simulink model "p4_v4"  (R2023b)
settings: Solver=VariableStepAuto  StartTime=0.0  StopTime=3600  RelTol=1e-3
values from neighbouring files (symbols this model uses):
  rps2rpm = 60/(2*pi())    [P4init.m]
undefined symbols (not defined in the file or in its folder): batData, carData, motorData
libraries: slpidlib x1
settings Model: Creator=lpoir  LastModifiedBy=lpoir

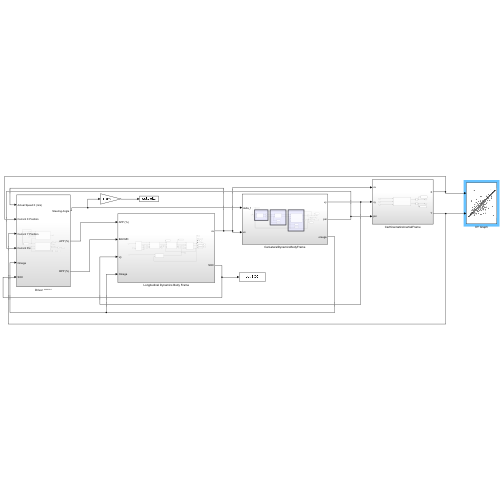
[thumbnail: Simulink's stored preview of the top-level diagram]
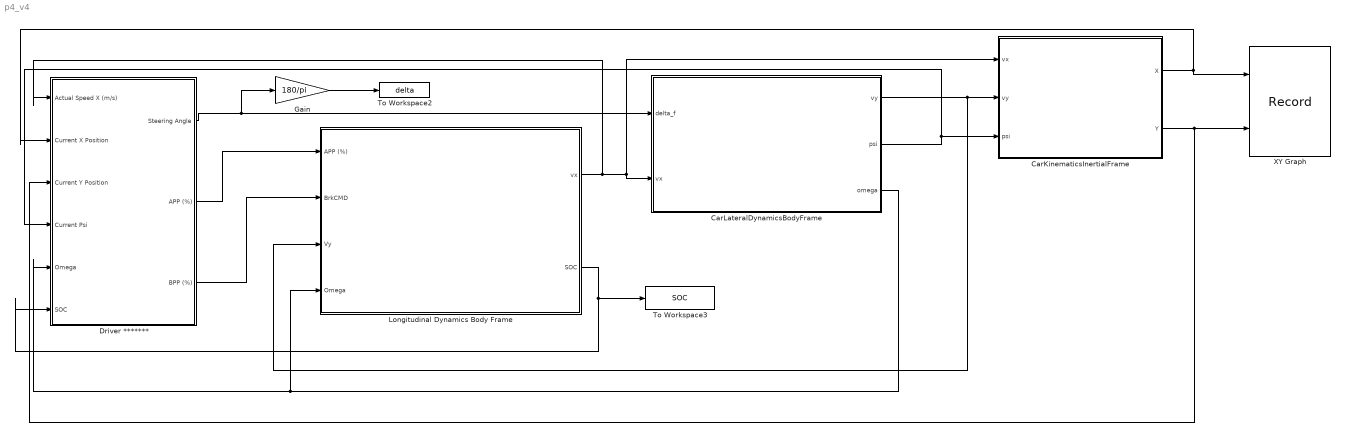
== system p4_v4 ==
  CarKinematicsInertialFrame : Subsystem
  CarLateralDynamicsBodyFrame : Subsystem
  Driver ******* : Subsystem
  Gain : Gain  Gain=180/pi
  Longitudinal Dynamics Body Frame : Subsystem
  To Workspace2 : ToWorkspace  VariableName=delta  SaveFormat=Timeseries  SampleTime=-1
  To Workspace3 : ToWorkspace  VariableName=SOC  SaveFormat=Timeseries  SampleTime=-1
  XY Graph : Record  FileSettingsInternal="{\"entries\":[{\"content\":{\"excelSettings\":{\"content\":{},\"type\":\"Streamout.ExcelSettings\"}},\"type\":\"Streamout.FileSettingStorage\",\"uuid\":\"\"}],\"packageUris\":[\"http:\\/\\/schema.mathworks.com\\/mf0\\/streamout_blocks\\/R2020a\"],\"version\":\"1.0\"}"  Layout=[1 1]  SignalsInternal="{\"entries\":[{\"content\":{\"signals\":[{\"content\":{\"blockPath\":[],\"dimensions\":[1],\"domain\":\"\",\"lineColor\":\"#a2142f\",\"plots\":[1],\"port\":1,\"sid\":[\"\"],\"signalID\":167009,\"signalName\":\"CarKinematicsInertialFrame:1\"},\"type\":\"RecordBlkView.Signal\",\"uuid\":\"\"},{\"content\":{\"blockPath\":[],\"dimensions\":[1],\"domain\":\"\",\"lineColor\":\"#139fff\",\"plots\":[1],\"port\":2,\"sid\":[\"\"],\"signalID\":167013,\"signalName\":\"CarKinematicsInertialFrame:2\"},\"type\":\"RecordBlkView.Signal\",\"uuid\":\"\"}]},\"type\":\"RecordBlkView.InputSignals\",\"uuid\":\"\"}],\"packageUris\":[\"http:\\/\\/schema.mathworks.com\\/mf0\\/streamout_blocks\\/R2020a\"],\"version\":\"1.0\"}"  VisualizationBindings="{\"xyplotplugin\":{\"info\":[{\"series\":[{\"bindingParametersList\":[{\"parameter\":\"X-Axis\",\"signalID\":167009,\"signalName\":\"CarKinematicsInertialFrame:1\"},{\"parameter\":\"Y-Axis\",\"signalID\":167013,\"signalName\":\"CarKinematicsInertialFrame:2\"}],\"seriesID\":48033}],\"subplotID\":1}]}}"  CompatibilityTag=XY
  wires:
  CarKinematicsInertialFrame/1(X) -> XY Graph/1, Driver *******/2(Current X Position)
  CarKinematicsInertialFrame/2(Y) -> XY Graph/2, Driver *******/3(Current Y Position)
  CarLateralDynamicsBodyFrame/2(psi) -> Driver *******/4("Current Psi "), CarKinematicsInertialFrame/3(psi)
  Longitudinal Dynamics Body Frame/1(vx) -> Driver *******/1(Actual Speed X (m/s)), CarKinematicsInertialFrame/1(vx), CarLateralDynamicsBodyFrame/2(vx)
  CarLateralDynamicsBodyFrame/3(omega) -> Longitudinal Dynamics Body Frame/4(Omega), Driver *******/5(Omega)
  Driver *******/1(Steering Angle) -> Gain/1, CarLateralDynamicsBodyFrame/1(delta_f)
  CarLateralDynamicsBodyFrame/1(vy) -> Longitudinal Dynamics Body Frame/3(Vy), CarKinematicsInertialFrame/2(vy)
  Driver *******/2(APP (%)) -> Longitudinal Dynamics Body Frame/1(APP (%))
  Driver *******/3(BPP (%)) -> Longitudinal Dynamics Body Frame/2("BrkCMD ")
  Longitudinal Dynamics Body Frame/2(SOC) -> To Workspace3/1, Driver *******/6(SOC)
  Gain/1 -> To Workspace2/1

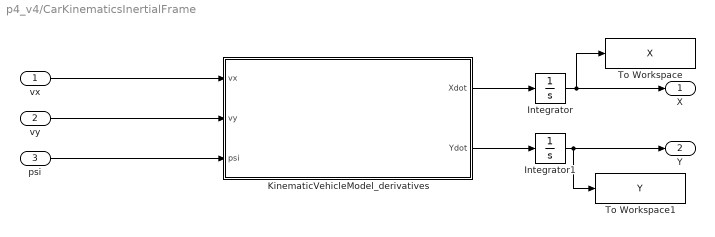
== system p4_v4/CarKinematicsInertialFrame ==
  vx : Inport
  vy : Inport  Port=2
  psi : Inport  Port=3
  Integrator : Integrator  InitialCondition=carData.init.X0
  Integrator1 : Integrator  InitialCondition=carData.init.Y0
  KinematicVehicleModel_derivatives : MATLAB Function  TreatAsAtomicUnit=on  mask{obj=carData}
      mask prompts: obj "obj structure"
  To Workspace : ToWorkspace  VariableName=X  SaveFormat=Timeseries  SampleTime=-1
  To Workspace1 : ToWorkspace  VariableName=Y  SaveFormat=Timeseries  SampleTime=-1
  X : Outport
  Y : Outport  Port=2
  wires:
  KinematicVehicleModel_derivatives/1(Xdot) -> Integrator/1
  KinematicVehicleModel_derivatives/2(Ydot) -> Integrator1/1
  Integrator/1 -> To Workspace/1, X/1
  Integrator1/1 -> To Workspace1/1, Y/1
  vx/1 -> KinematicVehicleModel_derivatives/1(vx)
  vy/1 -> KinematicVehicleModel_derivatives/2(vy)
  psi/1 -> KinematicVehicleModel_derivatives/3(psi)

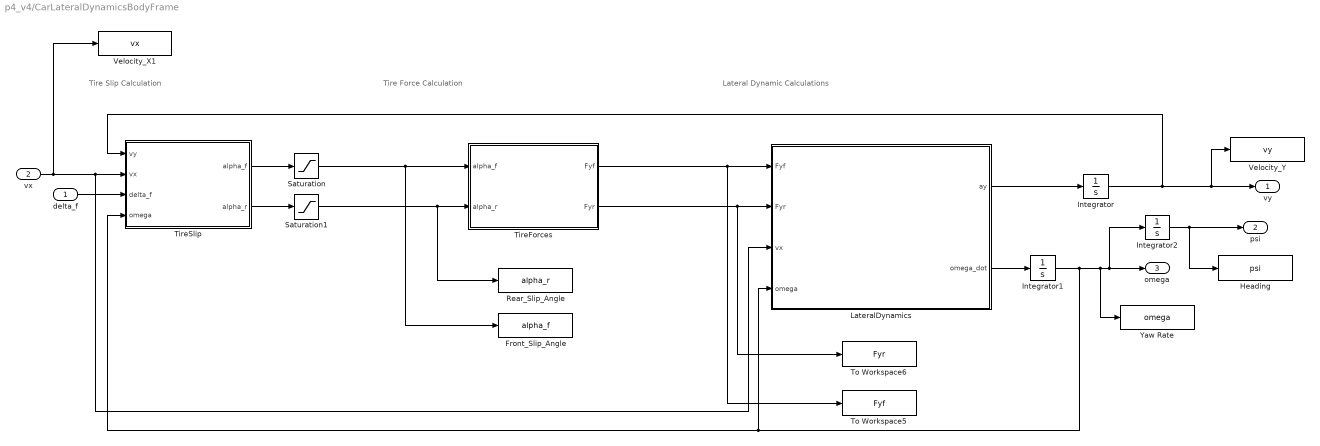
== system p4_v4/CarLateralDynamicsBodyFrame ==
  note: Tire Slip Calculation
  note: Tire Force Calculation
  note: Lateral Dynamic Calculations
  delta_f : Inport
  vx : Inport  Port=2
  Front_Slip_Angle : ToWorkspace  VariableName=alpha_f  SaveFormat=Timeseries  SampleTime=-1
  Heading : ToWorkspace  VariableName=psi  SaveFormat=Timeseries  SampleTime=-1
  Integrator : Integrator  InitialCondition=carData.init.vy0
  Integrator1 : Integrator  InitialCondition=carData.init.omega0
  Integrator2 : Integrator  InitialCondition=carData.init.psi0
  LateralDynamics : MATLAB Function  TreatAsAtomicUnit=on  mask{obj=carData}
      mask prompts: obj "obj structure"
  Rear_Slip_Angle : ToWorkspace  VariableName=alpha_r  SaveFormat=Timeseries  SampleTime=-1
  Saturation : Saturate  UpperLimit=carData.maxAlpha  LowerLimit=-carData.maxAlpha
  Saturation1 : Saturate  UpperLimit=carData.maxAlpha  LowerLimit=-carData.maxAlpha
  TireForces : MATLAB Function  TreatAsAtomicUnit=on  mask{obj=carData}
      mask prompts: obj "obj structure"
  TireSlip : MATLAB Function  TreatAsAtomicUnit=on  mask{obj=carData}
      mask prompts: obj "obj structure"
  To Workspace5 : ToWorkspace  VariableName=Fyf  SaveFormat=Timeseries  SampleTime=-1
  To Workspace6 : ToWorkspace  VariableName=Fyr  SaveFormat=Timeseries  SampleTime=-1
  Velocity_X1 : ToWorkspace  VariableName=vx  SaveFormat=Timeseries  SampleTime=-1
  Velocity_Y : ToWorkspace  VariableName=vy  SaveFormat=Timeseries  SampleTime=-1
  Yaw Rate : ToWorkspace  VariableName=omega  SaveFormat=Timeseries  SampleTime=-1
  vy : Outport
  psi : Outport  Port=2
  omega : Outport  Port=3
  wires:
  LateralDynamics/1(ay) -> Integrator/1
  Integrator/1 -> vy/1, Velocity_Y/1, TireSlip/1(vy)
  LateralDynamics/2(omega_dot) -> Integrator1/1
  Integrator1/1 -> Integrator2/1, omega/1, Yaw Rate/1, LateralDynamics/4(omega), TireSlip/4(omega)
  TireSlip/1(alpha_f) -> Saturation/1
  TireSlip/2(alpha_r) -> Saturation1/1
  TireForces/1(Fyf) -> LateralDynamics/1(Fyf), To Workspace5/1
  TireForces/2(Fyr) -> LateralDynamics/2(Fyr), To Workspace6/1
  Saturation/1 -> TireForces/1(alpha_f), Front_Slip_Angle/1
  Saturation1/1 -> TireForces/2(alpha_r), Rear_Slip_Angle/1
  vx/1 -> Velocity_X1/1, TireSlip/2(vx), LateralDynamics/3(vx)
  delta_f/1 -> TireSlip/3(delta_f)
  Integrator2/1 -> Heading/1, psi/1

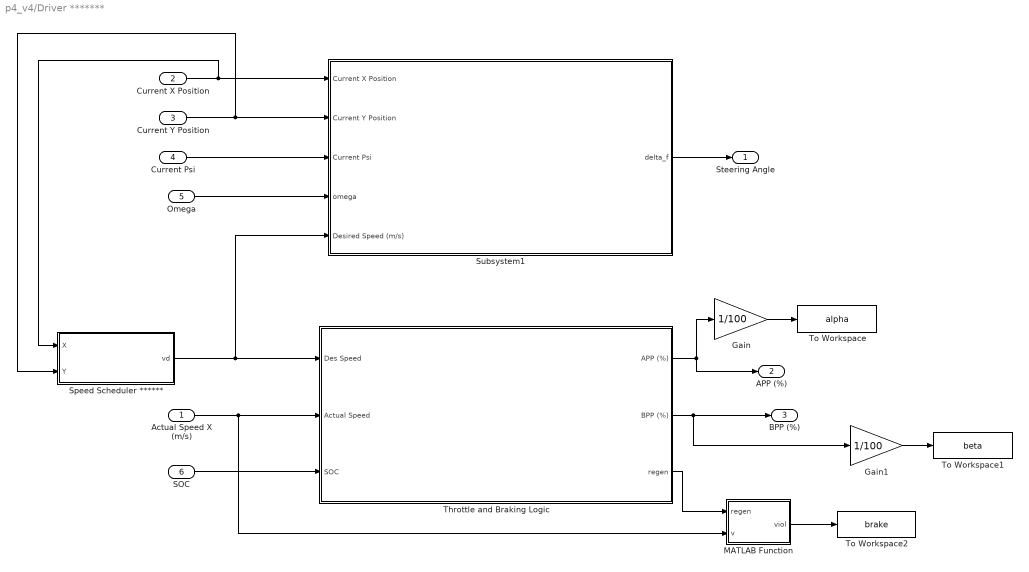
== system p4_v4/Driver ******* ==
  Actual Speed X (m/s) : Inport
  Current X Position : Inport  Port=2
  Current Y Position : Inport  Port=3
  "Current Psi " : Inport  Port=4
  Omega : Inport  Port=5
  SOC : Inport  Port=6
  Gain : Gain  Gain=1/100
  Gain1 : Gain  Gain=1/100
  MATLAB Function : MATLAB Function  TreatAsAtomicUnit=on
  Speed Scheduler ****** : MATLAB Function  TreatAsAtomicUnit=on
  Subsystem1 : Subsystem
  Throttle and Braking Logic : Subsystem
  To Workspace : ToWorkspace  VariableName=alpha  SaveFormat=Timeseries  SampleTime=-1
  To Workspace1 : ToWorkspace  VariableName=beta  SaveFormat=Timeseries  SampleTime=-1
  To Workspace2 : ToWorkspace  VariableName=brake  SaveFormat=Timeseries  SampleTime=-1
  Steering Angle : Outport
  APP (%) : Outport  Port=2
  BPP (%) : Outport  Port=3
  wires:
  Actual Speed X (m/s)/1 -> MATLAB Function/2(v), Throttle and Braking Logic/2(Actual Speed)
  SOC/1 -> Throttle and Braking Logic/3(SOC)
  Current X Position/1 -> Speed Scheduler ******/1(X), Subsystem1/1(Current X Position)
  Current Y Position/1 -> Speed Scheduler ******/2(Y), Subsystem1/2(Current Y Position)
  "Current Psi "/1 -> Subsystem1/3(Current Psi)
  Omega/1 -> Subsystem1/4(omega)
  Speed Scheduler ******/1(vd) -> Subsystem1/5(Desired Speed (m/s)), Throttle and Braking Logic/1("Des Speed ")
  Subsystem1/1(delta_f) -> Steering Angle/1
  Throttle and Braking Logic/1(APP (%)) -> Gain/1, APP (%)/1
  Throttle and Braking Logic/2(BPP (%)) -> Gain1/1, BPP (%)/1
  Gain/1 -> To Workspace/1
  Gain1/1 -> To Workspace1/1
  Throttle and Braking Logic/3(regen) -> MATLAB Function/1(regen)
  MATLAB Function/1(viol) -> To Workspace2/1

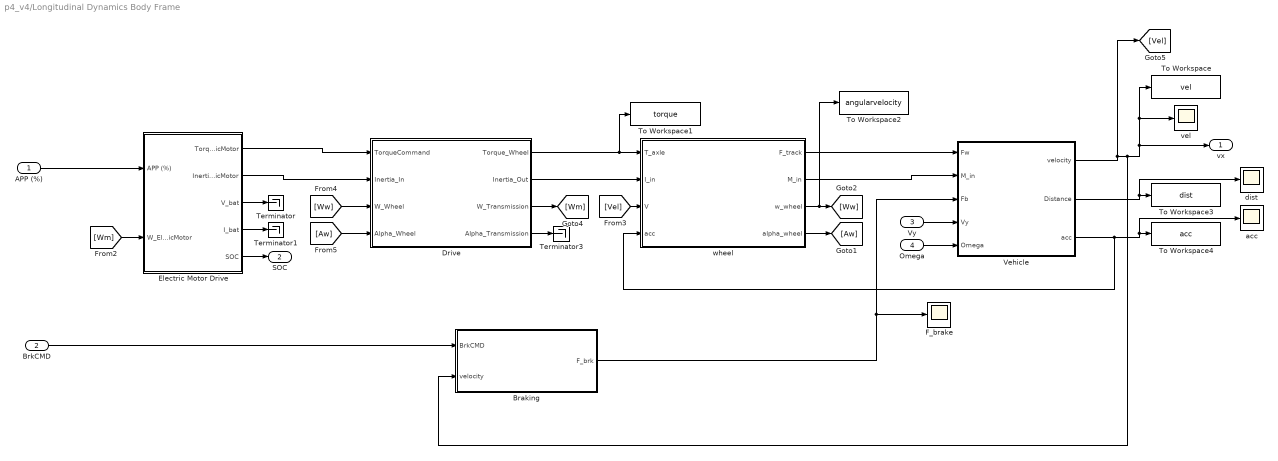
== system p4_v4/Longitudinal Dynamics Body Frame ==
  APP (%) : Inport
  "BrkCMD " : Inport  Port=2
  Vy : Inport  Port=3
  Omega : Inport  Port=4
  Braking : Subsystem
  Drive : Subsystem
  Electric Motor Drive : Subsystem  TreatAsAtomicUnit=on
  F_brake : Scope
  Terminator : Terminator
  Terminator1 : Terminator
  Terminator3 : Terminator
  To Workspace : ToWorkspace  VariableName=vel  SaveFormat=Timeseries  SampleTime=-1
  To Workspace1 : ToWorkspace  VariableName=torque  SaveFormat=Timeseries  SampleTime=-1
  To Workspace2 : ToWorkspace  VariableName=angularvelocity  SaveFormat=Timeseries  SampleTime=-1
  To Workspace3 : ToWorkspace  VariableName=dist  SaveFormat=Timeseries  SampleTime=-1
  To Workspace4 : ToWorkspace  VariableName=acc  SaveFormat=Timeseries  SampleTime=-1
  Vehicle : Subsystem
  acc : Scope
  dist : Scope
  vel : Scope
  "wheel " : Subsystem
  vx : Outport
  SOC : Outport  Port=2
  wires:
  Vehicle/1("velocity ") -> vel/1, To Workspace/1, vx/1, Braking/2("velocity "), [Vel]
  Electric Motor Drive/2(Inertia_ElectricMotor) -> Drive/2(Inertia_In)
  Drive/3(W_Transmission) -> [Wm]
  Electric Motor Drive/5(SOC) -> SOC/1
  Drive/2(Inertia_Out) -> "wheel "/2(I_in)
  [Aw] -> Drive/4(Alpha_Wheel)
  "wheel "/1(F_track) -> Vehicle/1("Fw ")
  Vehicle/2("Distance ") -> dist/1, To Workspace3/1
  [Ww] -> Drive/3(W_Wheel)
  "wheel "/2(M_in) -> Vehicle/2("M_in ")
  Drive/1(Torque_Wheel) -> "wheel "/1(T_axle), To Workspace1/1
  [Vel] -> "wheel "/3(V)
  Electric Motor Drive/4(I_bat) -> Terminator1/1
  [Wm] -> Electric Motor Drive/2(W_ElectricMotor)
  Electric Motor Drive/1(Torque_ElectricMotor) -> Drive/1(TorqueCommand)
  Vehicle/3(acc) -> acc/1, To Workspace4/1, "wheel "/4(acc)
  "BrkCMD "/1 -> Braking/1("BrkCMD ")
  Braking/1("F_brk ") -> F_brake/1, Vehicle/3("Fb ")
  "wheel "/4(alpha_wheel) -> [Aw]
  "wheel "/3(w_wheel) -> To Workspace2/1, [Ww]
  Drive/4(Alpha_Transmission) -> Terminator3/1
  Electric Motor Drive/3(V_bat) -> Terminator/1
  APP (%)/1 -> Electric Motor Drive/1(APP (%))
  Vy/1 -> Vehicle/4(Vy)
  Omega/1 -> Vehicle/5(Omega)

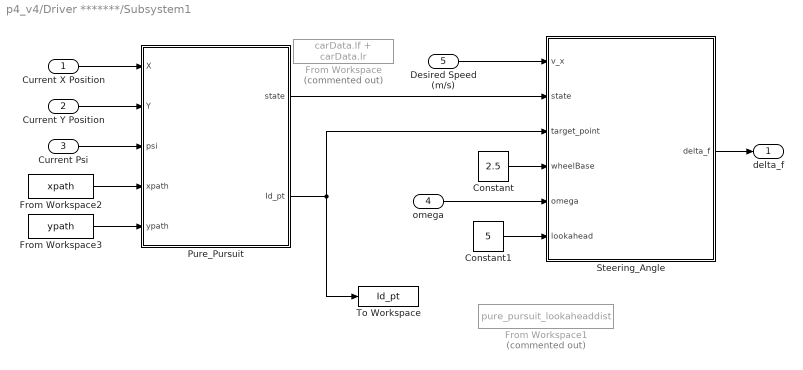
== system p4_v4/Driver *******/Subsystem1 ==
  Current X Position : Inport
  Current Y Position : Inport  Port=2
  Current Psi : Inport  Port=3
  omega : Inport  Port=4
  Desired Speed (m/s) : Inport  Port=5
  Constant : Constant  Value=2.5
  Constant1 : Constant  Value=5
  From Workspace : FromWorkspace  Commented=on  VariableName=carData.lf + carData.lr
  From Workspace1 : FromWorkspace  Commented=on  VariableName=pure_pursuit_lookaheaddist  OutDataTypeStr=single
  From Workspace2 : FromWorkspace  VariableName=xpath
  From Workspace3 : FromWorkspace  VariableName=ypath
  Pure_Pursuit : MATLAB Function  TreatAsAtomicUnit=on
  Steering_Angle : MATLAB Function  TreatAsAtomicUnit=on
  To Workspace : ToWorkspace  VariableName=Id_pt  SaveFormat=Timeseries  SampleTime=-1
  delta_f : Outport
  wires:
  Current X Position/1 -> Pure_Pursuit/1(X)
  Current Y Position/1 -> Pure_Pursuit/2(Y)
  Current Psi/1 -> Pure_Pursuit/3(psi)
  Pure_Pursuit/2(Id_pt) -> Steering_Angle/3(target_point), To Workspace/1
  Pure_Pursuit/1(state) -> Steering_Angle/2(state)
  Steering_Angle/1(delta_f) -> delta_f/1
  omega/1 -> Steering_Angle/5(omega)
  Desired Speed (m/s)/1 -> Steering_Angle/1(v_x)
  Constant/1 -> Steering_Angle/4(wheelBase)
  From Workspace2/1 -> Pure_Pursuit/4(xpath)
  From Workspace3/1 -> Pure_Pursuit/5(ypath)
  Constant1/1 -> Steering_Angle/6(lookahead)

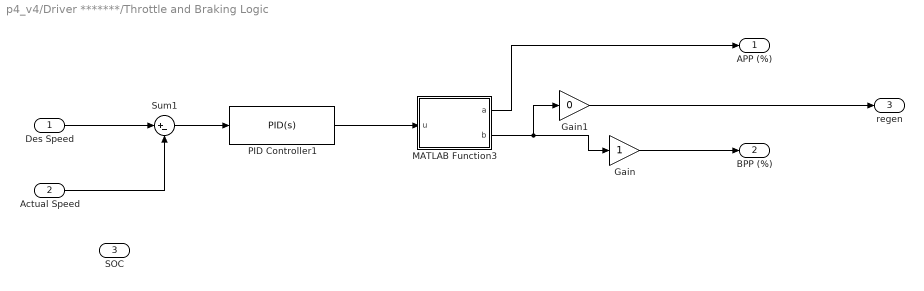
== system p4_v4/Driver *******/Throttle and Braking Logic ==
  "Des Speed " : Inport
  Actual Speed : Inport  Port=2
  SOC : Inport  Port=3
  Gain : Gain
  Gain1 : Gain  Gain=0
  MATLAB Function3 : MATLAB Function  TreatAsAtomicUnit=on
  PID Controller1 : slpidlib/PID Controller  Controller=PID  Form=Parallel  TimeDomain=Continuous-time  UseExternalTs=off  SampleTime=-1  IntegratorMethod=Forward Euler  FilterMethod=Forward Euler  ControllerParametersSource=internal  P=0.5  I=0  UseKiTs=off  D=0  N=100  UseFilter=on  TunerSelectOption=Transfer Function Based (PID Tuner App)  InitialConditionSource=internal  InitialConditionForIntegrator=0  InitialConditionForFilter=0  DifferentiatorICPrevScaledInput=0  ExternalReset=none  TrackingMode=off  Kt=1  LimitOutput=on  SatLimitsSource=internal  UpperSaturationLimit=1  LowerSaturationLimit=-1  LinearizeAsGain=off  AntiWindupMode=none  Kb=1  LimitIntegrator=off  UpperIntegratorSaturationLimit=inf  LowerIntegratorSaturationLimit=-inf  POutMin=[]  POutMax=[]  IOutMin=[]  IOutMax=[]  DOutMin=[]  DOutMax=[]  NOutMin=[]  NOutMax=[]  SumOutMin=[]  SumOutMax=[]  SaturationOutMin=[]  SaturationOutMax=[]  PParamMin=[]  PParamMax=[]  IParamMin=[]  IParamMax=[]  DParamMin=[]  DParamMax=[]  NParamMin=[]  NParamMax=[]  KbParamMin=[]  KbParamMax=[]  KtParamMin=[]  KtParamMax=[]  KbOutMin=[]  KbOutMax=[]  KtOutMin=[]  KtOutMax=[]  IntegratorOutMin=[]  IntegratorOutMax=[]  FilterOutMin=[]  FilterOutMax=[]  SumI1OutMin=[]  SumI1OutMax=[]  SumI2OutMin=[]  SumI2OutMax=[]  SumI3OutMin=[]  SumI3OutMax=[]  SumI4OutMin=[]  SumI4OutMax=[]  SumDOutMin=[]  SumDOutMax=[]  DifferentiatorOutMin=[]  DifferentiatorOutMax=[]  FilterDiffOutCoefMin=[]  FilterDiffOutCoefMax=[]  ReciprocalOutMin=[]  ReciprocalOutMax=[]  SumDenOutMin=[]  SumDenOutMax=[]  SumNumOutMin=[]  SumNumOutMax=[]  DivideOutMin=[]  DivideOutMax=[]  UdiffTsProdOutMin=[]  UdiffTsProdOutMax=[]  NTsProdOutMin=[]  NTsProdOutMax=[]  UintegralTsProdOutMin=[]  UintegralTsProdOutMax=[]  UngainTsProdOutMin=[]  UngainTsProdOutMax=[]  ClampingZeroOutDataTypeStr=Inherit: Inherit via back propagation  ClampingZeroOutMin=[]  ClampingZeroOutMax=[]  FilterDenConstantOutDataTypeStr=Inherit: Inherit via back propagation  FilterDenConstantOutMin=[]  FilterDenConstantOutMax=[]  PCopyOutDataTypeStr=Inherit: Inherit via back propagation  PCopyOutMin=[]  PCopyOutMax=[]  NCopyOutDataTypeStr=Inherit: Inherit via back propagation  NCopyOutMin=[]  NCopyOutMax=[]  IntegratorContinuousStateAttributes=''  IntegratorStateMustResolveToSignalObject=off  IntegratorRTWStateStorageClass=Auto  FilterContinuousStateAttributes=''  FilterStateMustResolveToSignalObject=off  FilterRTWStateStorageClass=Auto  ParallelPVariant=InternalParameters  IdealPVariant=Disabled  IVariant=InternalParameters  DVariant=InternalParameters  IntegratorVariant=Continuous  SatVariant=Enabled  AWVariant=Passthrough  PCopyVariant=Disabled  TRVariant=Disabled  FdbkBlocksVariant=Forward  IdealPFdbkVariant=Disabled  SatFdbkVariant=Disabled  DerivativeFilterVariant=ContFilter  NVariant=InternalParameters  NCopyVariant=Disabled  FilterICVariant=InternalICsFilter  IntegratorICVariant=InternalICs  ExternalResetVariant=Disabled  TRSumVariant=Passthrough  SumFdbkVariant=Disabled  SumVariant=Sum_PID  TsampFilterVariant=InternalTs  TsampNgainVariant=Passthrough  TsampIntegralVariant=Disabled_SignalSpec  ExternalSaturationOutDataTypeStr=Inherit: Same as second input
  Sum1 : Sum  Inputs=|+-
  APP (%) : Outport
  BPP (%) : Outport  Port=2
  regen : Outport  Port=3
  wires:
  "Des Speed "/1 -> Sum1/1
  MATLAB Function3/2(b) -> Gain1/1, Gain/1
  Actual Speed/1 -> Sum1/2
  Sum1/1 -> PID Controller1/1
  PID Controller1/1 -> MATLAB Function3/1(u)
  Gain/1 -> BPP (%)/1
  Gain1/1 -> regen/1
  MATLAB Function3/1(a) -> APP (%)/1

== system p4_v4/Longitudinal Dynamics Body Frame/Braking ==
  "BrkCMD " : Inport
  "velocity " : Inport  Port=2
  Gain1 : Gain  Gain=10000*carData.r
  MATLAB Function : MATLAB Function  TreatAsAtomicUnit=on
  MATLAB Function1 : MATLAB Function  Commented=on  TreatAsAtomicUnit=on
  "F_brk " : Outport  VectorParamsAs1DForOutWhenUnconnected=off
  wires:
  "BrkCMD "/1 -> Gain1/1
  Gain1/1 -> MATLAB Function/1(u)
  MATLAB Function/1(y) -> "F_brk "/1
  "velocity "/1 -> MATLAB Function/2(v)

== system p4_v4/Longitudinal Dynamics Body Frame/Drive ==
  TorqueCommand : Inport
  Inertia_In : Inport  Port=2
  W_Wheel : Inport  Port=3
  Alpha_Wheel : Inport  Port=4
  Gain : Gain  Gain=1500
  Torque_Wheel : Outport
  Inertia_Out : Outport  Port=2
  W_Transmission : Outport  Port=3
  Alpha_Transmission : Outport  Port=4
  wires:
  TorqueCommand/1 -> Gain/1
  Gain/1 -> Torque_Wheel/1
  Inertia_In/1 -> Inertia_Out/1
  W_Wheel/1 -> W_Transmission/1
  Alpha_Wheel/1 -> Alpha_Transmission/1

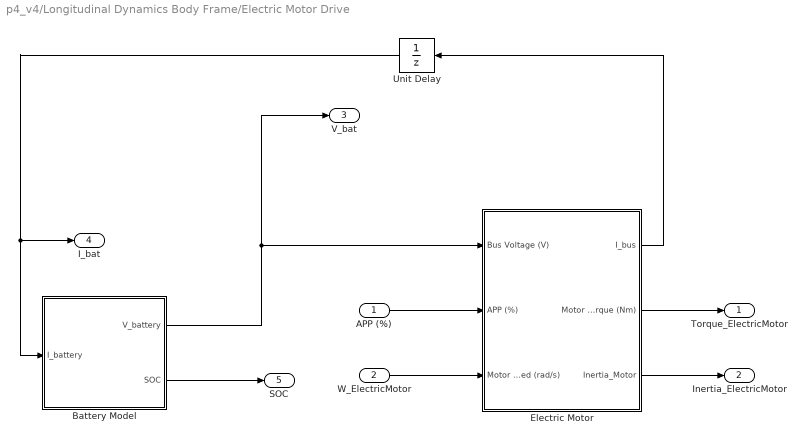
== system p4_v4/Longitudinal Dynamics Body Frame/Electric Motor Drive ==
  APP (%) : Inport
  W_ElectricMotor : Inport  Port=2
  Battery Model : Subsystem  TreatAsAtomicUnit=on
  Electric Motor : Subsystem  TreatAsAtomicUnit=on
  Unit Delay : UnitDelay  SampleTime=-1  HasFrameUpgradeWarning=on
  Torque_ElectricMotor : Outport
  Inertia_ElectricMotor : Outport  Port=2
  V_bat : Outport  Port=3
  I_bat : Outport  Port=4
  SOC : Outport  Port=5
  wires:
  APP (%)/1 -> Electric Motor/2(APP (%))
  W_ElectricMotor/1 -> Electric Motor/3(Motor Speed (rad/s))
  Battery Model/1(V_battery) -> Electric Motor/1(Bus Voltage (V)), V_bat/1
  Electric Motor/2(Motor Torque (Nm)) -> Torque_ElectricMotor/1
  Electric Motor/3(Inertia_Motor) -> Inertia_ElectricMotor/1
  Battery Model/2(SOC) -> SOC/1
  Electric Motor/1(I_bus) -> Unit Delay/1
  Unit Delay/1 -> Battery Model/1(I_battery), I_bat/1

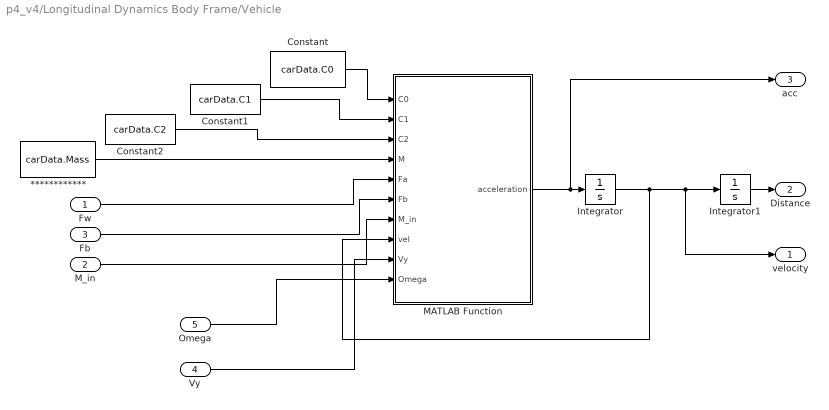
== system p4_v4/Longitudinal Dynamics Body Frame/Vehicle ==
  "Fw " : Inport
  "M_in " : Inport  Port=2
  "Fb " : Inport  Port=3
  Vy : Inport  Port=4
  Omega : Inport  Port=5
  ************ : Constant  Value=carData.Mass
  Constant : Constant  Value=carData.C0
  Constant1 : Constant  Value=carData.C1
  Constant2 : Constant  Value=carData.C2
  Integrator : Integrator  LimitOutput=on  LowerSaturationLimit=0
  Integrator1 : Integrator
  MATLAB Function : MATLAB Function  TreatAsAtomicUnit=on
  "velocity " : Outport  VectorParamsAs1DForOutWhenUnconnected=off
  "Distance " : Outport  Port=2  VectorParamsAs1DForOutWhenUnconnected=off
  acc : Outport  Port=3
  wires:
  MATLAB Function/1(acceleration) -> acc/1, Integrator/1
  "Fw "/1 -> MATLAB Function/5(Fa)
  "Fb "/1 -> MATLAB Function/6(Fb)
  Integrator/1 -> MATLAB Function/8(vel), "velocity "/1, Integrator1/1
  Integrator1/1 -> "Distance "/1
  "M_in "/1 -> MATLAB Function/7(M_in)
  Vy/1 -> MATLAB Function/9(Vy)
  Omega/1 -> MATLAB Function/10(Omega)
  ************/1 -> MATLAB Function/4(M)
  Constant2/1 -> MATLAB Function/3(C2)
  Constant1/1 -> MATLAB Function/2(C1)
  Constant/1 -> MATLAB Function/1(C0)

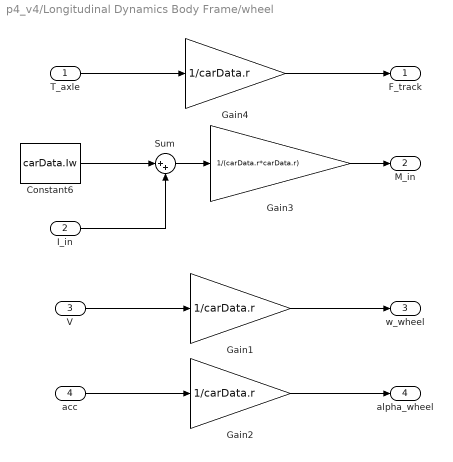
== system p4_v4/Longitudinal Dynamics Body Frame/wheel  ==
  T_axle : Inport
  I_in : Inport  Port=2
  V : Inport  Port=3
  acc : Inport  Port=4
  Constant6 : Constant  Value=carData.Iw
  Gain1 : Gain  Gain=1/carData.r
  Gain2 : Gain  Gain=1/carData.r
  Gain3 : Gain  Gain=1/(carData.r*carData.r)
  Gain4 : Gain  Gain=1/carData.r
  Sum : Sum  Inputs=|++
  F_track : Outport
  M_in : Outport  Port=2
  w_wheel : Outport  Port=3
  alpha_wheel : Outport  Port=4
  wires:
  T_axle/1 -> Gain4/1
  Constant6/1 -> Sum/1
  I_in/1 -> Sum/2
  Gain4/1 -> F_track/1
  V/1 -> Gain1/1
  Gain1/1 -> w_wheel/1
  acc/1 -> Gain2/1
  Gain2/1 -> alpha_wheel/1
  Gain3/1 -> M_in/1
  Sum/1 -> Gain3/1

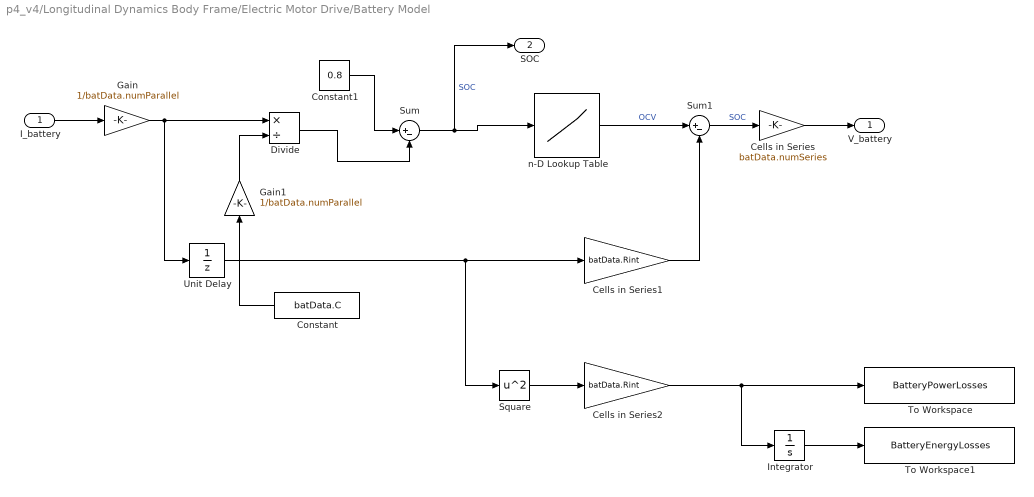
== system p4_v4/Longitudinal Dynamics Body Frame/Electric Motor Drive/Battery Model ==
  I_battery : Inport
  Cells in Series : Gain  Gain=batData.numSeries
  Cells in Series1 : Gain  Gain=batData.Rint
  Cells in Series2 : Gain  Gain=batData.Rint
  Constant : Constant  Value=batData.C
  Constant1 : Constant  Value=0.8
  Divide : Product  Inputs=*/
  Gain : Gain  Gain=1/batData.numParallel
  Gain1 : Gain  Gain=1/batData.numParallel
  Integrator : Integrator
  Square : Math  Operator=square
  Sum : Sum  Inputs=|+-
  Sum1 : Sum  Inputs=|+-
  To Workspace : ToWorkspace  VariableName=BatteryPowerLosses  SaveFormat=Timeseries  SampleTime=-1
  To Workspace1 : ToWorkspace  VariableName=BatteryEnergyLosses  SaveFormat=Timeseries  SampleTime=-1
  Unit Delay : UnitDelay  SampleTime=-1  HasFrameUpgradeWarning=on
  n-D Lookup Table : Lookup_n-D  NumberOfTableDimensions=1  BreakpointsForDimension1=batData.SOC  BreakpointsForDimension3=[5, 7]  Table=batData.OCV  InternalRulePriority=Speed  RndMeth=Simplest
  V_battery : Outport
  SOC : Outport  Port=2
  wires:
  I_battery/1 -> Gain/1
  Gain/1 -> Unit Delay/1, Divide/1
  Gain1/1 -> Divide/2
  Constant/1 -> Gain1/1
  Constant1/1 -> Sum/1
  Divide/1 -> Sum/2
  Sum/1 -> SOC/1, n-D Lookup Table/1  "SOC"
  n-D Lookup Table/1 -> Sum1/1  "OCV"
  Cells in Series/1 -> V_battery/1
  Sum1/1 -> Cells in Series/1  "SOC"
  Cells in Series1/1 -> Sum1/2
  Square/1 -> Cells in Series2/1
  Cells in Series2/1 -> Integrator/1, To Workspace/1
  Integrator/1 -> To Workspace1/1
  Unit Delay/1 -> Square/1, Cells in Series1/1

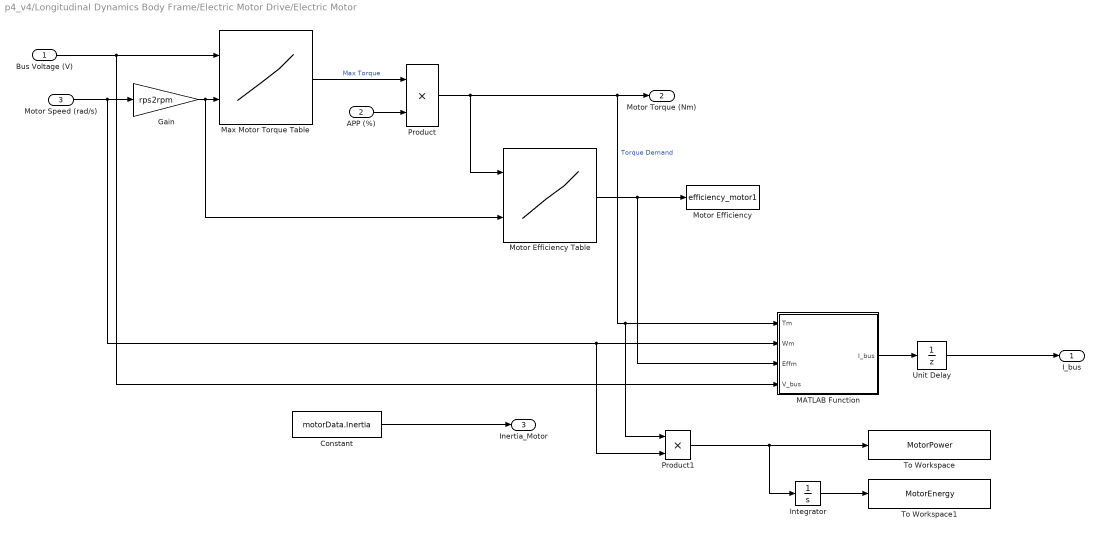
== system p4_v4/Longitudinal Dynamics Body Frame/Electric Motor Drive/Electric Motor ==
  Bus Voltage (V) : Inport
  APP (%) : Inport  Port=2
  Motor Speed (rad/s) : Inport  Port=3
  Constant : Constant  Value=motorData.Inertia
  Gain : Gain  Gain=rps2rpm
  Integrator : Integrator
  MATLAB Function : MATLAB Function  TreatAsAtomicUnit=on
  Max Motor Torque Table : Lookup_n-D  BreakpointsForDimension1=motorData.vbus  BreakpointsForDimension2=motorData.rpm  BreakpointsForDimension3=[5, 7]  Table=motorData.maxtorque  InternalRulePriority=Speed  RndMeth=Simplest
      settings: InputPortMap=u0,u1
  Motor Efficiency : ToWorkspace  VariableName=efficiency_motor1  SaveFormat=Timeseries  SampleTime=-1
  Motor Efficiency Table : Lookup_n-D  BreakpointsForDimension1=motorData.eta_torque  BreakpointsForDimension2=motorData.eta_speed  BreakpointsForDimension3=[5, 7]  Table=motorData.eta_val  InternalRulePriority=Speed  RndMeth=Simplest
      settings: InputPortMap=u0,u1
  Product : Product
  Product1 : Product
  To Workspace : ToWorkspace  VariableName=MotorPower  SaveFormat=Timeseries  SampleTime=-1
  To Workspace1 : ToWorkspace  VariableName=MotorEnergy  SaveFormat=Timeseries  SampleTime=-1
  Unit Delay : UnitDelay  SampleTime=-1  HasFrameUpgradeWarning=on
  I_bus : Outport
  Motor Torque (Nm) : Outport  Port=2
  Inertia_Motor : Outport  Port=3
  wires:
  Constant/1 -> Inertia_Motor/1
  APP (%)/1 -> Product/2
  Max Motor Torque Table/1 -> Product/1  "Max Torque"
  Product/1 -> Motor Efficiency Table/1, Product1/1, MATLAB Function/1(Tm), Motor Torque (Nm)/1  "Torque Demand"
  Gain/1 -> Motor Efficiency Table/2, Max Motor Torque Table/2
  Motor Speed (rad/s)/1 -> Product1/2, MATLAB Function/2(Wm), Gain/1
  Motor Efficiency Table/1 -> MATLAB Function/3(Effm), Motor Efficiency/1
  Integrator/1 -> To Workspace1/1
  Product1/1 -> Integrator/1, To Workspace/1
  MATLAB Function/1(I_bus) -> Unit Delay/1
  Unit Delay/1 -> I_bus/1
  Bus Voltage (V)/1 -> MATLAB Function/4(V_bus), Max Motor Torque Table/1

== matlab function p4_v4/Longitudinal Dynamics Body Frame/Braking/MATLAB Function1 ==
  data: regen input; viol output; v input
function viol = violfcn(regen, v)
    speed = (3600/1600)*v;
    if speed < 5
        regen_vio = 0;
        if regen == regen_vio
            viol = 0;
        else
            viol = 1;
        end

    elseif speed == 25
        regen_vio = 0.95;
        if regen == regen_vio
            viol = 0;
        else
            viol = 1;
        end

    elseif v > 25
        regen_vio = 0.95;
        if regen == regen_vio
            viol = 0;
        else
            viol = 1;
        end
    else
        regen_vio = ((0.95/20)*speed) - 0.2375;
        if regen == regen_vio
            viol = 0;
        else
            viol = 1;
        end
    end

== matlab function p4_v4/Driver *******/Throttle and Braking Logic/MATLAB Function3 ==
  data: u input; a output; b output
function [a,b] = fcn(u)

if u>0
    acc=u;
    brk=0;
elseif u<0
    acc=0;
    brk=-u;
else
    acc=0;
    brk=0;
end
a= acc;
b= brk;

== matlab function p4_v4/Driver *******/Subsystem1/Pure_Pursuit ==
  data: X input; state output; Y input; psi input; Id_pt output; xpath input; ypath input
function [state, Id_pt] = pure_pursuit(X,Y,psi,xpath,ypath)

state = [X,Y,psi];

num_points = length(xpath);

xpath_update = xpath(1:num_points);
ypath_update = ypath(1:num_points);

num_points = length(xpath_update);

dist_from_waypoints_sqr = (xpath_update - X).^2 + (ypath_update - Y).^2;
dist_from_waypoints = sqrt(dist_from_waypoints_sqr);

[~, idx] = min(dist_from_waypoints);

targ_idx = idx + 5;
if targ_idx > num_points
    targ_idx = 1;
end

x_targ = xpath_update(targ_idx);
y_targ = ypath_update(targ_idx);

Id_pt = [x_targ, y_targ, psi];

== matlab function p4_v4/Driver *******/MATLAB Function ==
  data: regen input; viol output; v input
function viol = violfcn(regen, v)
    speed = (3600/1600)*v;
    if speed < 5
        regen_vio = 0;
        if regen == regen_vio
            viol = 0;
        else
            viol = 1;
        end

    elseif speed == 25
        regen_vio = 0.95;
        if regen == regen_vio
            viol = 0;
        else
            viol = 1;
        end

    elseif v > 25
        regen_vio = 0.95;
        if regen == regen_vio
            viol = 0;
        else
            viol = 1;
        end
    else
        regen_vio = ((0.95/20)*speed) - 0.2375;
        if regen == regen_vio
            viol = 0;
        else
            viol = 1;
        end
    end

== matlab function p4_v4/Driver *******/Speed Scheduler ****** ==
  data: X input; vd output; Y input
function vd = fcn(X, Y)

if X > 0 && X < 900
    vd = 15;
else
    vd = 10;
end

== matlab function p4_v4/CarLateralDynamicsBodyFrame/LateralDynamics ==
  data: Fyf input; Fyr input size=1; vx input; omega input; ay output; obj parameter; omega_dot output
function [ay, omega_dot] = fcn(Fyf, Fyr, vx, omega, obj)

Fy = Fyf + Fyr;
ay = Fy / obj.Mass - omega * vx;
        
M  = Fyf * obj.lf - Fyr * obj.lr;        
omega_dot = M / obj.Inertia;        

end

== matlab function p4_v4/Longitudinal Dynamics Body Frame/Vehicle/MATLAB Function ==
  data: C0 input; acceleration output; C1 input; C2 input; M input; Fa input; Fb input; M_in input; vel input; Vy input; Omega input
function acceleration   = vehicle(C0,C1,C2,M,Fa,Fb,M_in, vel, Vy, Omega)

acceleration = (((Fa-Fb))-(C0+ C1*vel + C2*(vel)^2))/(M+M_in) + Vy * Omega;

== matlab function p4_v4/CarKinematicsInertialFrame/KinematicVehicleModel_derivatives ==
  data: vx input; vy input; psi input size=1; Xdot output; Ydot output
function [Xdot, Ydot] = fcn(vx, vy, psi)
    temp = TF(psi) * [vx;vy]; 
    Xdot = temp(1);
    Ydot = temp(2);
  
end

function y = TF(psi)
    y = [cos(psi), -sin(psi); sin(psi), cos(psi)];
end

== matlab function p4_v4/Longitudinal Dynamics Body Frame/Electric Motor Drive/Electric Motor/MATLAB Function ==
  data: Tm input; I_bus output; Wm input; Effm input; V_bus input
function I_bus = fcn(Tm,Wm,Effm,V_bus)

%I_bus = (Tm*Wm/Effm)/V_bus;

Pm=Tm*Wm;
sgnPm = Pm/(abs(Pm)+0.001);
I_bus = ( (Pm) * (Effm)^(sgnPm) ) / V_bus;

== matlab function p4_v4/CarLateralDynamicsBodyFrame/TireForces ==
  data: alpha_f input; alpha_r input; Fyf output; obj parameter; Fyr output
function [Fyf, Fyr] = fcn(alpha_f, alpha_r, obj)

Fyf = min(obj.Fyfmax,obj.Calpha_f * alpha_f);
Fyr = min(obj.Fyrmax, obj.Calpha_r * alpha_r);
end

== matlab function p4_v4/CarLateralDynamicsBodyFrame/TireSlip ==
  data: vy input size=1; vx input; delta_f input size=1; omega input; alpha_f output; obj parameter; alpha_r output
function [alpha_f, alpha_r] = fcn(vy,  vx, delta_f, omega, obj)


if abs(vx)> obj.vx_threshold1
      alpha_f = delta_f - (vy + omega * obj.lf) / vx;
      alpha_r = - (vy - omega * obj.lr) / vx;
else
      alpha_f = 0;
      alpha_r = 0;
end



end

== matlab function p4_v4/Longitudinal Dynamics Body Frame/Braking/MATLAB Function ==
  data: u input; y output; v input
function y = fcn(u,v)
%y =u*sign(v)
y = u * v/(abs(v)+0.001);
y = u;

== matlab function p4_v4/Driver *******/Subsystem1/Steering_Angle ==
  data: v_x input; delta_f output; state input; target_point input; wheelBase input; omega input; lookahead input
% INPUTS
%   v_x - actual velocity
%   state - current state of the vehicle
%   target_point - target point of the vehicle
%   omega - current yaw rate of the vehicle

% OUTPUTS
%   delta_f - the steering angle of the vehicle

function delta_f = latControl(v_x, state, target_point, wheelBase, omega, lookahead)

% current position of the vehicle
current_X = state(1);
current_Y = state(2);
current_psi = state(3);

% target position where we want the vehicle to go
targ_X = target_point(1);
targ_Y = target_point(2);
targ_psi = target_point(3);

alpha = atan2(targ_Y - current_Y, targ_X - current_X) - current_psi;
psi_dot_d = (2 * wheelBase * sin(alpha)) / lookahead;
delta_f = atan(psi_dot_d);
